simulink model "PB2_DCS_810698349"  (R2021b)
settings: Solver=VariableStepAuto  StartTime=0.0  StopTime=5  RelTol=1e-3
undefined symbols (not defined in the file or in its folder): C, Dd, G, Gd, H, Ts
settings Model: Creator=SinaK  LastModifiedBy=SinaK

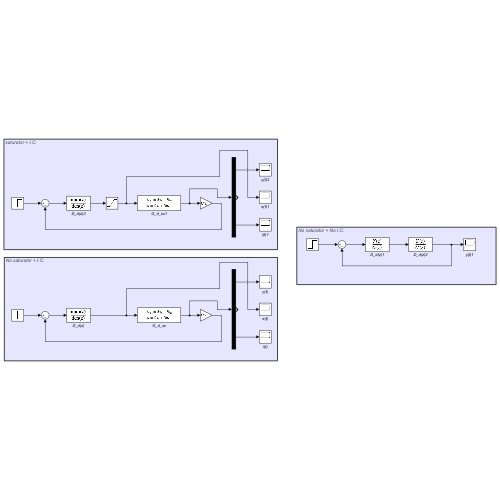
[thumbnail: Simulink's stored preview of the top-level diagram]
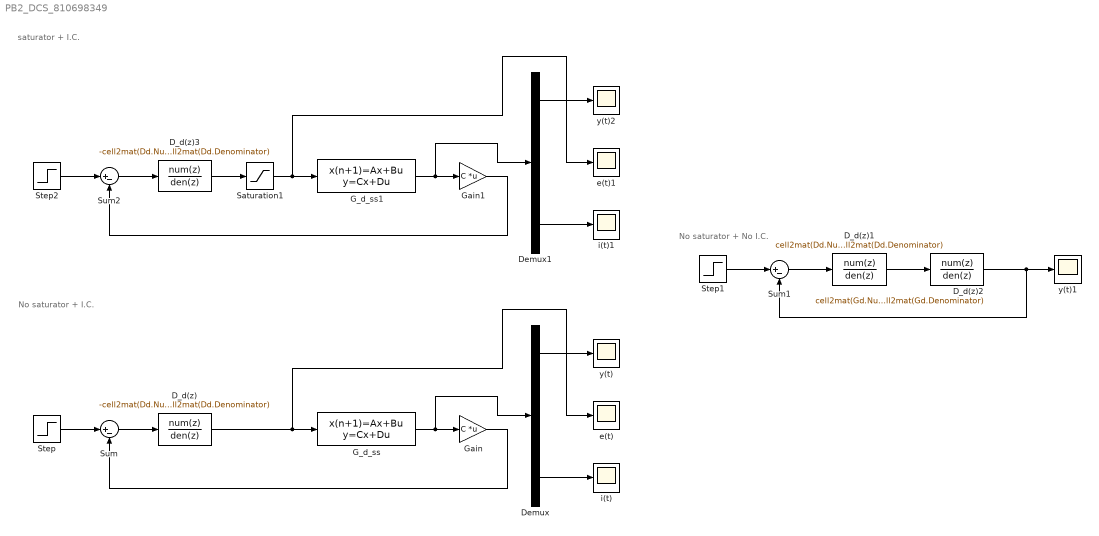
== system PB2_DCS_810698349 ==
  note: No saturator + No I.C.
  note: No saturator + I.C.
  note: saturator + I.C.
  D_d(z) : DiscreteTransferFcn  Numerator=-cell2mat(Dd.Numerator)  Denominator=cell2mat(Dd.Denominator)  SampleTime=Ts
  D_d(z)1 : DiscreteTransferFcn  Numerator=cell2mat(Dd.Numerator)  Denominator=cell2mat(Dd.Denominator)  SampleTime=Ts
  D_d(z)2 : DiscreteTransferFcn  Numerator=cell2mat(Gd.Numerator)  Denominator=cell2mat(Gd.Denominator)  SampleTime=Ts
  D_d(z)3 : DiscreteTransferFcn  Numerator=-cell2mat(Dd.Numerator)  Denominator=cell2mat(Dd.Denominator)  SampleTime=Ts
  Demux : Demux  Outputs=3
  Demux1 : Demux  Outputs=3
  G_d_ss : DiscreteStateSpace  A=G  B=H  C=eye(3)  D=[0;0;0]  InitialCondition=[12 0 0]  SampleTime=Ts
  G_d_ss1 : DiscreteStateSpace  A=G  B=H  C=eye(3)  D=[0;0;0]  InitialCondition=[12 0 0]  SampleTime=Ts
  Gain : Gain  Gain=C  Multiplication=Matrix(K*u)
  Gain1 : Gain  Gain=C  Multiplication=Matrix(K*u)
  Saturation1 : Saturate  UpperLimit=12  LowerLimit=0
  Step : Step  Time=0  After=10  SampleTime=Ts
  Step1 : Step  Time=0  After=10  SampleTime=Ts
  Step2 : Step  Time=0  After=10  SampleTime=Ts
  Sum : Sum  Inputs=|+-
  Sum1 : Sum  Inputs=|+-
  Sum2 : Sum  Inputs=|+-
  e(t) : Scope
  e(t)1 : Scope
  i(t) : Scope
  i(t)1 : Scope
  y(t) : Scope
  y(t)1 : Scope
  y(t)2 : Scope
  wires:
  Sum/1 -> D_d(z)/1
  Step/1 -> Sum/1
  Gain/1 -> Sum/2
  G_d_ss/1 -> Demux/1, Gain/1
  Demux/1 -> y(t)/1
  Demux/3 -> i(t)/1
  Sum1/1 -> D_d(z)1/1
  Step1/1 -> Sum1/1
  D_d(z)1/1 -> D_d(z)2/1
  D_d(z)2/1 -> Sum1/2, y(t)1/1
  D_d(z)/1 -> G_d_ss/1, e(t)/1
  D_d(z)3/1 -> Saturation1/1
  Sum2/1 -> D_d(z)3/1
  Gain1/1 -> Sum2/2
  Step2/1 -> Sum2/1
  Demux1/3 -> i(t)1/1
  G_d_ss1/1 -> Demux1/1, Gain1/1
  Demux1/1 -> y(t)2/1
  Saturation1/1 -> G_d_ss1/1, e(t)1/1
